simulink model "simulink_projesi"  (R2019a)
settings: Solver=VariableStepAuto  StartTime=0.0  StopTime=10.0  RelTol=1e-3
settings Model: Creator=PC_393_ADMIN  LastModifiedBy=PC_393_ADMIN

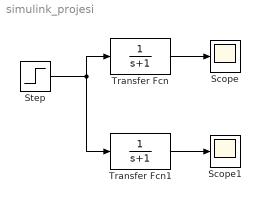
== system simulink_projesi ==
  Scope : Scope
  Scope1 : Scope
  Step : Step  SampleTime=0
  Transfer Fcn : TransferFcn  Denominator=[1 1]
  Transfer Fcn1 : TransferFcn  Denominator=[1 1]
  wires:
  Transfer Fcn/1 -> Scope/1
  Step/1 -> Transfer Fcn1/1, Transfer Fcn/1
  Transfer Fcn1/1 -> Scope1/1
